simulink model "eas4710_waypoint_block"  (R2024b)
settings: Solver=ode45  StartTime=0.0  StopTime=30.0  RelTol=1e-3  EnableMultiTasking=on
values from neighbouring files (symbols this model uses):
  Aact = [-20.2 0;0 -20.1]    [AutoPilot.m]
  Aele = -10    [AutoPilot.m]
  Alatd = [-0.2008       0.2807       0         0.7823      -0.4131     0 ... (first row only)    [AutoPilot.m]
  Along = [-0.0507         20.6655      -9.8100     -0.7028     0 0 ... (first row only)    [AutoPilot.m]
  Atau = -1    [AutoPilot.m]
  Bact = [20.2 0;0 20.2] * Beta    [AutoPilot.m]
  Bele = 10 * Beta    [AutoPilot.m]
  Blatd = [.00012049 .00032897;0 0;0 0;-.1031578 .020987;-.002133 -.010715;0 0]    [AutoPilot.m]
  Blong = [0;0;0;-.019781;0;0]    [AutoPilot.m]
  Btau = 1    [AutoPilot.m]
  Cact = [-1 0;0 -1]    [AutoPilot.m]
  Cele = -1    [AutoPilot.m]
  Clatd = [0 0 0 0 0 1;57 0 0 0 0 0;0 0 57 0 0 0 ... (first row only)    [AutoPilot.m]
  Clong = [0 0 0 0 0 1;0 0 0 0 1 0;1 0 0 0 0 0 ... (first row only)    [AutoPilot.m]
  Ctau = -1    [AutoPilot.m]
  Dact = [0 0;0 0]    [AutoPilot.m]
  Dele = 0    [AutoPilot.m]
  Dlatd = zeros(6,2)    [AutoPilot.m]
  Dlong = zeros(6,1)    [AutoPilot.m]
  Dtau = 1    [AutoPilot.m]
  Kd = Gains(1)    [AutoPilot.m]
  Kh = Gains(2)    [AutoPilot.m]
  Kk = Gains(3)    [AutoPilot.m]
  Kp = Gains(6)    [AutoPilot.m]
  Kq = Gains(4)    [AutoPilot.m]
  Kr = Gains(7)    [AutoPilot.m]
  Kt = Gains(5)    [AutoPilot.m]
  V = 500    [AutoPilot.m]
undefined symbols (not defined in the file or in its folder): Aalt, Balt, Calt, Dalt
settings Model: Creator=rick  LastModifiedBy=austi
settings SolverCC: AlgebraicLoopSolver=TrustRegion
settings DataIOCC: LimitDataPoints=on  SaveFormat=Array  SignalLoggingSaveFormat=ModelDataLogs  ReturnWorkspaceOutputs=off
settings OptimizationCC: ExpressionDepthLimit=2147483647  InitFltsAndDblsToZero=on  LifeSpan=inf
settings DebuggingCC: SaveWithParameterizedLinksMsg=none  UnderspecifiedInitializationDetection=Classic  MergeDetectMultiDrivingBlocksExec=none  SignalResolutionControl=TryResolveAllWithWarning  MultiTaskDSMMsg=warning  MultiTaskCondExecSysMsg=none  FcnCallInpInsideContextMsg=warning  UnconnectedInputMsg=warning  UnconnectedOutputMsg=warning  UnconnectedLineMsg=warning  StateNameClashWarn=warning  SFUnexpectedBacktrackingDiag=warning  SFNoUnconditionalDefaultTransitionDiag=warning  SFExecutionAtInitializationDiag=none  ArithmeticOperatorsInVariantConditions=warning
settings HardwareCC: ProdBitPerPointer=32  ProdBitPerSizeT=32  ProdBitPerPtrDiffT=32  ProdLargestAtomicFloat=None  ProdIntDivRoundTo=Undefined  ProdEndianess=Unspecified  ProdWordSize=32  ProdHWDeviceType=32-bit Generic
settings ModelReferenceCC: EnableRefExpFcnMdlSchedulingChecks=on  PropagateSignalLabelsOutOfModel=off
settings SFSimCC: SimUseLocalCustomCode=off  CustomCodeUndefinedFunction=UseInterfaceOnly
settings RTWCC: RTWUseLocalCustomCode=off  GPUComputeCapability=3.5
settings CodeAppCC: StateflowObjectComments=on
settings GRTTargetCC: TargetFcnLib=ansi_tfl_tmw.mat  TargetLangStandard=C89/C90 (ANSI)  CombineOutputUpdateFcns=off  GRTInterface=on
settings ConfigComp: CovMetricSettings=dw  CovSaveCumulativeToWorkspaceVar=on  CovSaveSingleToWorkspaceVar=on  CovExternalEMLEnable=off

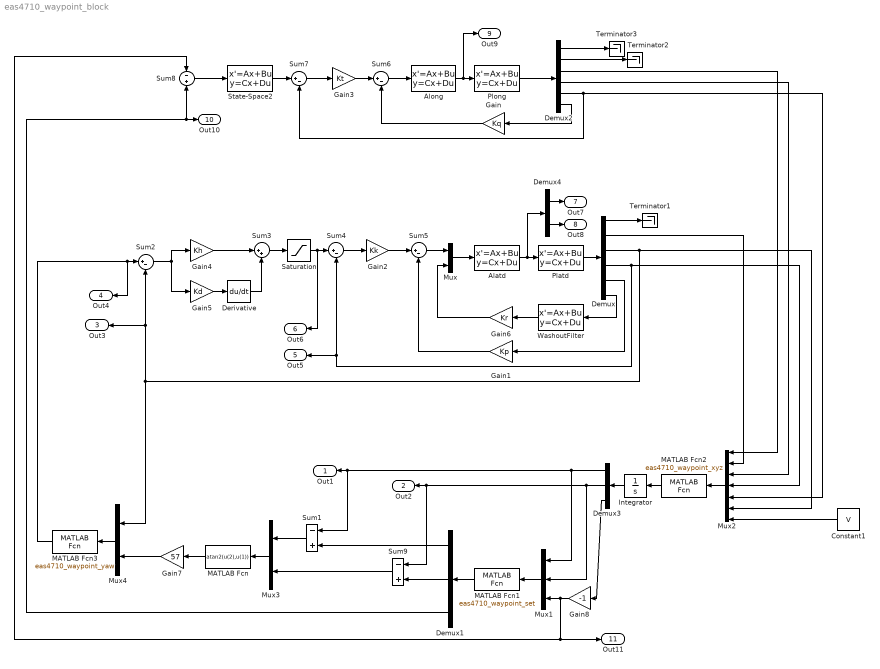
== system eas4710_waypoint_block ==
  Alatd : StateSpace  A=Aact  B=Bact  C=Cact  D=Dact  InitialCondition=0
  Along : StateSpace  A=Aele  B=Bele  C=Cele  D=Dele  InitialCondition=0
  Constant1 : Constant  Value=V
  Demux : Demux  Outputs=6
  Demux1 : Demux  Outputs=3
  Demux2 : Demux  Outputs=6
  Demux3 : Demux  Outputs=3
  Demux4 : Demux  Outputs=2
  Derivative : Derivative
  Gain : Gain  Gain=Kq
  Gain1 : Gain  Gain=Kp
  Gain2 : Gain  Gain=Kk
  Gain3 : Gain  Gain=Kt
  Gain4 : Gain  Gain=Kh
  Gain5 : Gain  Gain=Kd
  Gain6 : Gain  Gain=Kr
  Gain7 : Gain  Gain=57
  Gain8 : Gain  Gain=-1
  Integrator : Integrator
  MATLAB Fcn : MATLABFcn  MATLABFcn=atan2(u(2),u(1))
  MATLAB Fcn1 : MATLABFcn  MATLABFcn=eas4710_waypoint_set
  MATLAB Fcn2 : MATLABFcn  MATLABFcn=eas4710_waypoint_xyz
  MATLAB Fcn3 : MATLABFcn  MATLABFcn=eas4710_waypoint_yaw  OutputDimensions=1
  Mux : Mux  Inputs=2
  Mux1 : Mux  Inputs=3
  Mux2 : Mux  Inputs=7
  Mux3 : Mux  Inputs=2
  Mux4 : Mux  Inputs=2
  Platd : StateSpace  A=Alatd  B=Blatd  C=Clatd  D=Dlatd  InitialCondition=0
  Plong : StateSpace  A=Along  B=Blong  C=Clong  D=Dlong  InitialCondition=0
  Saturation : Saturate  UpperLimit=40  LowerLimit=-40
  State-Space2 : StateSpace  A=Aalt  B=Balt  C=Calt  D=Dalt  InitialCondition=0
  Sum1 : Sum  Inputs=-+
  Sum{2,4..7} (5 alike) : Sum  Inputs=|+-
  Sum3 : Sum  Inputs=|++
  Sum8 : Sum  Inputs=-+
  Sum9 : Sum  Inputs=-+
  Terminator1 : Terminator
  Terminator2 : Terminator
  Terminator3 : Terminator
  WashoutFilter : StateSpace  A=Atau  B=Btau  C=Ctau  D=Dtau  InitialCondition=0
  Out1 : Outport
  Out2 : Outport  Port=2
  Out3 : Outport  Port=3
  Out4 : Outport  Port=4
  Out5 : Outport  Port=5
  Out6 : Outport  Port=6
  Out7 : Outport  Port=7
  Out8 : Outport  Port=8
  Out9 : Outport  Port=9
  Out10 : Outport  Port=10
  Out11 : Outport  Port=11
  wires:
  Alatd/1 -> Platd/1, Demux4/1
  Platd/1 -> Demux/1
  Gain2/1 -> Sum5/1
  Mux/1 -> Alatd/1
  Sum5/1 -> Mux/1
  Gain4/1 -> Sum3/1
  Sum3/1 -> Saturation/1
  Demux/3 -> Mux2/6, Sum2/2, Out3/1, Mux4/1
  Sum2/1 -> Gain4/1, Gain5/1
  Derivative/1 -> Sum3/2
  Gain5/1 -> Derivative/1
  Sum4/1 -> Gain2/1
  Gain6/1 -> Mux/2
  WashoutFilter/1 -> Gain6/1
  Gain1/1 -> Sum5/2
  Sum9/1 -> Mux3/2
  Sum1/1 -> Mux3/1
  MATLAB Fcn1/1 -> Demux1/1
  Mux1/1 -> MATLAB Fcn1/1
  Saturation/1 -> Sum4/1, Out6/1
  Along/1 -> Plong/1, Out9/1
  Gain/1 -> Sum6/2
  Plong/1 -> Demux2/1
  Sum6/1 -> Along/1
  Gain3/1 -> Sum6/1
  Sum7/1 -> Gain3/1
  State-Space2/1 -> Sum7/1
  Sum8/1 -> State-Space2/1
  Demux2/6 -> Gain/1
  Demux2/5 -> Sum7/2, Mux2/5
  Demux/6 -> WashoutFilter/1
  Demux/5 -> Gain1/1
  Demux/4 -> Sum4/2, Out5/1, Mux2/4
  MATLAB Fcn2/1 -> Integrator/1
  Integrator/1 -> Demux3/1
  Mux2/1 -> MATLAB Fcn2/1
  Constant1/1 -> Mux2/7
  Demux2/3 -> Mux2/1
  Demux2/4 -> Mux2/3
  Demux/2 -> Mux2/2
  Demux2/1 -> Terminator3/1
  Demux/1 -> Terminator1/1
  Demux3/1 -> Mux1/1, Sum1/1, Out1/1
  Demux3/2 -> Mux1/2, Sum9/1, Out2/1
  Mux3/1 -> MATLAB Fcn/1
  Demux4/1 -> Out7/1
  Demux4/2 -> Out8/1
  Demux1/3 -> Sum8/2, Out10/1
  MATLAB Fcn/1 -> Gain7/1
  MATLAB Fcn3/1 -> Sum2/1, Out4/1
  Gain7/1 -> Mux4/2
  Mux4/1 -> MATLAB Fcn3/1
  Demux2/2 -> Terminator2/1
  Gain8/1 -> Mux1/3, Sum8/1, Out11/1
  Demux3/3 -> Gain8/1
  Demux1/2 -> Sum9/2
  Demux1/1 -> Sum1/2
